simulink model "FullVehicleModel_ABS_ESP"  (R2020a)
settings: Solver=ode23s  StartTime=0.0  StopTime=t_f  MaxStep=0.1  RelTol=1e-3
values from neighbouring files (symbols this model uses):
  acc_US_test = 0.1    [mainVehicleModel.m]
  auxiliary_data = getAuxiliaryDataStruct()    [mainVehicleModel.m]
  curv_akermann = 1/50.    (= 0.02)    [mainVehicleModel.m]
  init_conditions_data = getInitialConditionsDataStruct( V_init )    [mainVehicleModel.m]
  lambda_max = -0.055    [mainVehicleModel.m]
  lambda_min = -0.08    [mainVehicleModel.m]
  maneuver_flag = 4    [mainVehicleModel.m]
  t_brake = t_f+1    (= 111)    [mainVehicleModel.m]
  Tb_max = Fb_max*vehicle_data.rear_wheel.Rr    [mainVehicleModel.m]
  Tb_min = Fb_min*vehicle_data.rear_wheel.Rr    [mainVehicleModel.m]
  V_init = 50    [mainVehicleModel.m]
  vehicle_data = getVehicleDataStruct()    [mainVehicleModel.m]
undefined symbols (not defined in the file or in its folder): k, magnitude, sigbuilder_block
libraries: dspfdesign x1, simulink x1
settings Model: SimulationMode=accelerator  Creator=luca  LastModifiedBy=Pasquale Romano
settings DataIOCC: ReturnWorkspaceOutputs=off
settings DebuggingCC: ArithmeticOperatorsInVariantConditions=warning
settings SFSimCC: SimUseLocalCustomCode=off  CustomCodeUndefinedFunction=UseInterfaceOnly
settings RTWCC: RTWUseLocalCustomCode=off
settings CodeAppCC: StateflowObjectComments=on

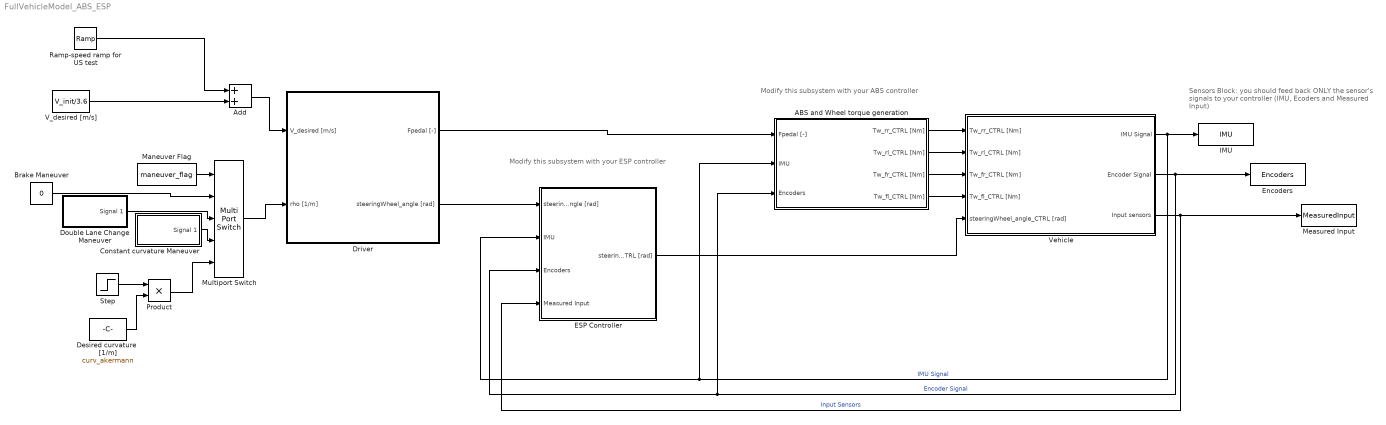
== system FullVehicleModel_ABS_ESP ==
  note: Modify this subsystem with your ABS controller
  note: Modify this subsystem with your ESP
      | controller
  note: Sensors Block: you should feed back ONLY
      | the sensor's signals to your controller
      | (IMU, Ecoders and Measured Input)
  ABS and Wheel torque generation : Subsystem
  Add : Sum
  Brake Maneuver : Constant  Value=0
  Constant curvature Maneuver : Subsystem  Tag=STV Subsys  LoadFcn=sigbuilder_block('load');  StartFcn=sigbuilder_block('start');  StopFcn=sigbuilder_block('stop');  ClipboardFcn=sigbuilder_block('clipboard');  mask(Sigbuilder block){tuvar=[0:10]}
      mask help: Simulink:masks:SigbuilderBlock_MD
      mask init:
      | if ~strcmp(get_param(bdroot(gcbh),'SimulationStatus'),'stopped') tuvar = sigbuilder_block('maskInit'); end
      settings: CopyFcn=sigbuilder_block('copy');  DeleteFcn=sigbuilder_block('delete');  ModelCloseFcn=sigbuilder_block('modelClose');  PreSaveFcn=sigbuilder_block('preSave');  PauseFcn=sigbuilder_block('pause');  ContinueFcn=sigbuilder_block('continue');  NameChangeFcn=sigbuilder_block('namechange');  OpenFcn=sigbuilder_block('open',[0 0 1319 754 ]);  CloseFcn=sigbuilder_block('close');
      mask Display: plot(0, 0, 100, 100,[2, 2, 32, 32, 2], [68, 8, 8, 68, 68],[32, 2], [38, 38], [32, 19, 2],[53, 60, 44], [32, 17, 17, 2],[16, 16, 31, 31]);txt = getActiveGroup(gcbh);text(2, 100, txt,'verticalAlignment', 'top');
  Desired curvature  [1/m] : Constant  Value=curv_akermann
  Double Lane Change Maneuver : Subsystem  Tag=STV Subsys  LoadFcn=sigbuilder_block('load');  StartFcn=sigbuilder_block('start');  StopFcn=sigbuilder_block('stop');  ClipboardFcn=sigbuilder_block('clipboard');  mask(Sigbuilder block){tuvar=[0:10]}
      mask help: Simulink:masks:SigbuilderBlock_MD
      mask init:
      | if ~strcmp(get_param(bdroot(gcbh),'SimulationStatus'),'stopped') tuvar = sigbuilder_block('maskInit'); end
      settings: CopyFcn=sigbuilder_block('copy');  DeleteFcn=sigbuilder_block('delete');  ModelCloseFcn=sigbuilder_block('modelClose');  PreSaveFcn=sigbuilder_block('preSave');  PauseFcn=sigbuilder_block('pause');  ContinueFcn=sigbuilder_block('continue');  NameChangeFcn=sigbuilder_block('namechange');  OpenFcn=sigbuilder_block('open',[0 0 1280 649 ]);  CloseFcn=sigbuilder_block('close');
      mask Display: plot(0, 0, 100, 100,[2, 2, 32, 32, 2], [68, 8, 8, 68, 68],[32, 2], [38, 38], [32, 19, 2],[53, 60, 44], [32, 17, 17, 2],[16, 16, 31, 31]);txt = getActiveGroup(gcbh);text(2, 100, txt,'verticalAlignment', 'top');
  Driver : Subsystem
  ESP Controller : Subsystem
  Encoders : ToWorkspace  VariableName=Encoders  SaveFormat=Timeseries  SampleTime=-1
  IMU : ToWorkspace  VariableName=IMU  SaveFormat=Timeseries  SampleTime=-1
  Maneuver Flag : Constant  Value=maneuver_flag
  Measured Input : ToWorkspace  VariableName=MeasuredInput  SaveFormat=Timeseries  SampleTime=-1
  Multiport Switch : MultiPortSwitch  Inputs=4
  Product : Product
  Ramp-speed ramp for US test : simulink/Sources/Ramp  slope=acc_US_test  start=Tstart_US_test  InitialOutput=0
  Step : Step  SampleTime=0
  V_desired [m/s] : Constant  Value=V_init/3.6
  Vehicle : Subsystem
  wires:
  Driver/1(Fpedal [-]) -> ABS and Wheel torque generation/1(Fpedal [-])
  Driver/2(steeringWheel_angle [rad]) -> ESP Controller/1(steeringWheel_angle [rad])
  Vehicle/1(IMU Signal) -> IMU/1, ABS and Wheel torque generation/2(IMU), ESP Controller/2(IMU)  "IMU Signal"
  Vehicle/2(Encoder Signal) -> Encoders/1, ABS and Wheel torque generation/3(Encoders), ESP Controller/3(Encoders)  "Encoder Signal"
  Vehicle/3(Input sensors) -> Measured Input/1, ESP Controller/4(Measured Input)  "Input Sensors"
  ESP Controller/1(steeringWheel_angle_CTRL [rad]) -> Vehicle/5(steeringWheel_angle_CTRL [rad])
  Double Lane Change Maneuver/1(Signal 1) -> Multiport Switch/3
  Constant curvature Maneuver/1(Signal 1) -> Multiport Switch/4
  Multiport Switch/1 -> Driver/2(rho [1/m])
  Brake Maneuver/1 -> Multiport Switch/2
  Maneuver Flag/1 -> Multiport Switch/1
  ABS and Wheel torque generation/4(Tw_fl_CTRL [Nm]) -> Vehicle/4(Tw_fl_CTRL [Nm])
  ABS and Wheel torque generation/3(Tw_fr_CTRL [Nm]) -> Vehicle/3(Tw_fr_CTRL [Nm])
  ABS and Wheel torque generation/2(Tw_rl_CTRL [Nm]) -> Vehicle/2(Tw_rl_CTRL [Nm])
  ABS and Wheel torque generation/1(Tw_rr_CTRL [Nm]) -> Vehicle/1(Tw_rr_CTRL [Nm])
  Desired curvature  [1/m]/1 -> Product/2
  Step/1 -> Product/1
  Product/1 -> Multiport Switch/5
  Ramp-speed ramp for US test/1 -> Add/1
  V_desired [m/s]/1 -> Add/2
  Add/1 -> Driver/1(V_desired [m/s])

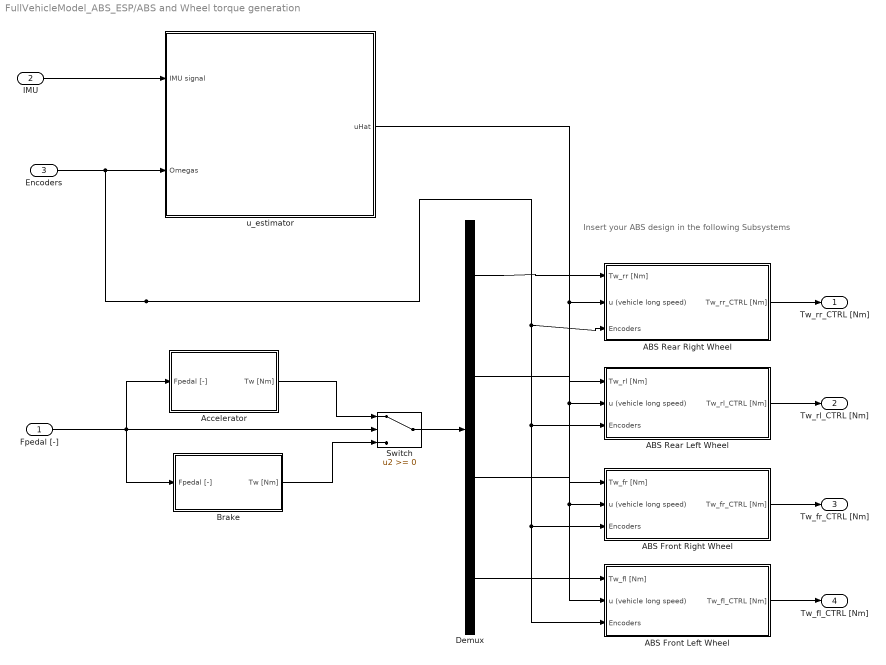
== system FullVehicleModel_ABS_ESP/ABS and Wheel torque generation ==
  note: Insert your ABS design in the
      | following Subsystems
  Fpedal [-] : Inport
  IMU : Inport  Port=2
  Encoders : Inport  Port=3
  ABS Front Left Wheel : Subsystem
  ABS Front Right Wheel : Subsystem
  ABS Rear Left Wheel : Subsystem
  ABS Rear Right Wheel : Subsystem
  Accelerator : Subsystem
  Brake : Subsystem
  Demux : Demux
  Switch : Switch
  u_estimator : Subsystem
  Tw_rr_CTRL [Nm] : Outport  VectorParamsAs1DForOutWhenUnconnected=off
  Tw_rl_CTRL [Nm] : Outport  Port=2  VectorParamsAs1DForOutWhenUnconnected=off
  Tw_fr_CTRL [Nm] : Outport  Port=3  VectorParamsAs1DForOutWhenUnconnected=off
  Tw_fl_CTRL [Nm] : Outport  Port=4  VectorParamsAs1DForOutWhenUnconnected=off
  wires:
  Demux/2 -> ABS Rear Left Wheel/1(Tw_rl [Nm])
  Switch/1 -> Demux/1
  Demux/1 -> ABS Rear Right Wheel/1(Tw_rr [Nm])
  Fpedal [-]/1 -> Brake/1(Fpedal [-]), Accelerator/1(Fpedal [-]), Switch/2
  ABS Rear Right Wheel/1(Tw_rr_CTRL [Nm]) -> Tw_rr_CTRL [Nm]/1
  Encoders/1 -> u_estimator/2(Omegas), ABS Rear Right Wheel/3(Encoders), ABS Front Left Wheel/3(Encoders), ABS Front Right Wheel/3(Encoders), ABS Rear Left Wheel/3(Encoders)
  ABS Rear Left Wheel/1(Tw_rl_CTRL [Nm]) -> Tw_rl_CTRL [Nm]/1
  Demux/3 -> ABS Front Right Wheel/1(Tw_fr [Nm])
  ABS Front Right Wheel/1(Tw_fr_CTRL [Nm]) -> Tw_fr_CTRL [Nm]/1
  Demux/4 -> ABS Front Left Wheel/1(Tw_fl [Nm])
  ABS Front Left Wheel/1(Tw_fl_CTRL [Nm]) -> Tw_fl_CTRL [Nm]/1
  Accelerator/1(Tw [Nm]) -> Switch/1
  Brake/1(Tw [Nm]) -> Switch/3
  IMU/1 -> u_estimator/1(IMU signal)
  u_estimator/1(uHat) -> ABS Front Right Wheel/2("u (vehicle long speed) "), ABS Front Left Wheel/2("u (vehicle long speed) "), ABS Rear Left Wheel/2("u (vehicle long speed) "), ABS Rear Right Wheel/2("u (vehicle long speed) ")

== system FullVehicleModel_ABS_ESP/Constant curvature Maneuver ==
  Demux : Demux  Tag=STV Demux  Outputs=1
      settings: DisplayOption=none
  FromWs : FromWorkspace  Tag=STV FromWs  VariableName=tuvar
      SigBuilderData=|
      | common.afterFinalStr = 'Extrapolate'
      | common.sampleTime = 0
      | dataSet.timeRange = [0 20]
      | dataSet.name = 'Group 1'
      | sbobj.Groups.Name = 'Group 1'
      | sbobj.Groups.Signals.Name = 'Signal 1'
      | sbobj.Groups.Signals.XData = [0 0.98 0.98 20]
      | sbobj.Groups.Signals.YData = [0 0 0.4 0.4]
      | sbobj.Groups.TimeRange = [0 20]
  Signal 1 : Outport  Tag=STV Outport  VectorParamsAs1DForOutWhenUnconnected=off
  wires:
  Demux/1 -> Signal 1/1
  FromWs/1 -> Demux/1

== system FullVehicleModel_ABS_ESP/Double Lane Change Maneuver ==
  Demux : Demux  Tag=STV Demux  Outputs=1
      settings: DisplayOption=none
  FromWs : FromWorkspace  Tag=STV FromWs  VariableName=tuvar
      SigBuilderData=|
      | common.afterFinalStr = 'Extrapolate'
      | common.sampleTime = 0
      | dataSet.timeRange = [0 10]
      | dataSet.name = 'Group 1'
      | sbobj.Groups.Name = 'Group 1'
      | sbobj.Groups.Signals.Name = 'Signal 1'
      | sbobj.Groups.Signals.XData = [0 1 1 1.5 1.5 1.6 1.6 2.1 2.1 3 3 3.5 3.5 3.7 3.7 4.2 4.2 10]
      | sbobj.Groups.Signals.YData = [0 0 0.5 0.5 0 0 -0.504 -0.504 0 0 -0.5 -0.5 0 0 0.5 0.5 0 0]
  Signal 1 : Outport  Tag=STV Outport  VectorParamsAs1DForOutWhenUnconnected=off
  wires:
  FromWs/1 -> Demux/1
  Demux/1 -> Signal 1/1

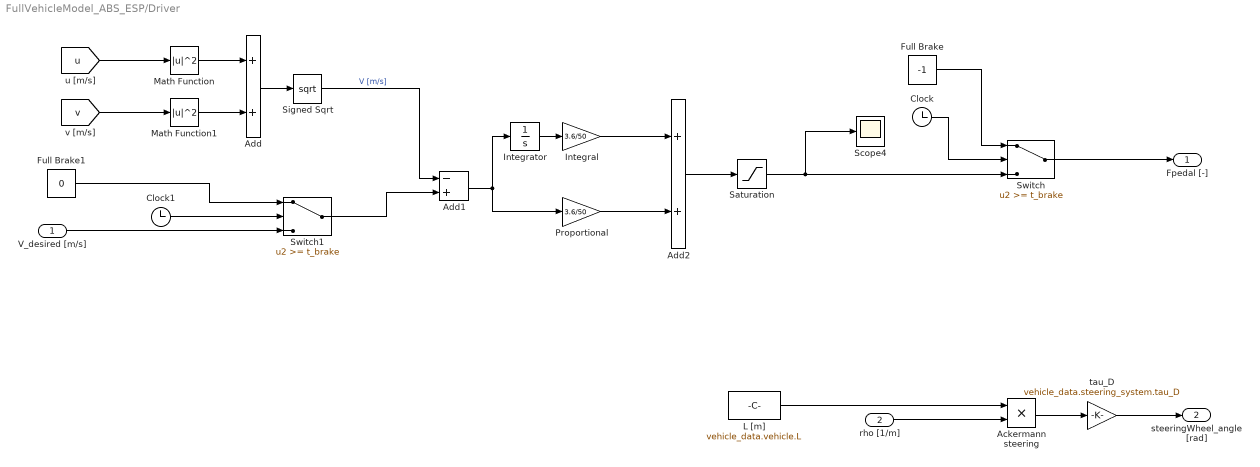
== system FullVehicleModel_ABS_ESP/Driver ==
  V_desired [m/s] : Inport
  rho [1/m] : Inport  Port=2
  Ackermann steering : Product  Inputs=**
  Add : Sum
  Add1 : Sum  Inputs=-+
  Add2 : Sum
  Clock : Clock
  Clock1 : Clock
  Full Brake : Constant  Value=-1
  Full Brake1 : Constant  Value=0
  Integral : Gain  Gain=3.6/50
  Integrator : Integrator
  L [m] : Constant  Value=vehicle_data.vehicle.L
  Math Function : Math  Operator=magnitude^2  SignedPower=on  SaturateOnIntegerOverflow=on
  Math Function1 : Math  Operator=magnitude^2  SignedPower=on  SaturateOnIntegerOverflow=on
  Proportional : Gain  Gain=3.6/50
  Saturation : Saturate  UpperLimit=1  LowerLimit=-1
  Scope4 : Scope
  Signed Sqrt : Sqrt  SaturateOnIntegerOverflow=on
  Switch : Switch  Threshold=t_brake
  Switch1 : Switch  Threshold=t_brake
  tau_D : Gain  Gain=vehicle_data.steering_system.tau_D
  Fpedal [-] : Outport  VectorParamsAs1DForOutWhenUnconnected=off
  steeringWheel_angle [rad] : Outport  Port=2  VectorParamsAs1DForOutWhenUnconnected=off
  wires:
  Proportional/1 -> Add2/2
  Add2/1 -> Saturation/1
  Integrator/1 -> Integral/1
  L [m]/1 -> Ackermann steering/1
  Add/1 -> Signed Sqrt/1
  Math Function1/1 -> Add/2
  Add1/1 -> Integrator/1, Proportional/1
  Signed Sqrt/1 -> Add1/1  "V [m/s]"
  Ackermann steering/1 -> tau_D/1
  Math Function/1 -> Add/1
  rho [1/m]/1 -> Ackermann steering/2
  Integral/1 -> Add2/1
  [u] -> Math Function/1
  [v] -> Math Function1/1
  V_desired [m/s]/1 -> Switch1/3
  Saturation/1 -> Switch/3, Scope4/1
  Full Brake1/1 -> Switch1/1
  Clock1/1 -> Switch1/2
  Full Brake/1 -> Switch/1
  Clock/1 -> Switch/2
  Switch/1 -> Fpedal [-]/1
  Switch1/1 -> Add1/2
  tau_D/1 -> steeringWheel_angle [rad]/1

== system FullVehicleModel_ABS_ESP/ESP Controller ==
  steeringWheel_angle [rad] : Inport
  IMU : Inport  Port=2
  Encoders : Inport  Port=3
  Measured Input : Inport  Port=4
  Terminator : Terminator
  Terminator1 : Terminator
  Terminator2 : Terminator
  steeringWheel_angle_CTRL [rad] : Outport  VectorParamsAs1DForOutWhenUnconnected=off
  wires:
  steeringWheel_angle [rad]/1 -> steeringWheel_angle_CTRL [rad]/1
  IMU/1 -> Terminator/1
  Encoders/1 -> Terminator1/1
  Measured Input/1 -> Terminator2/1

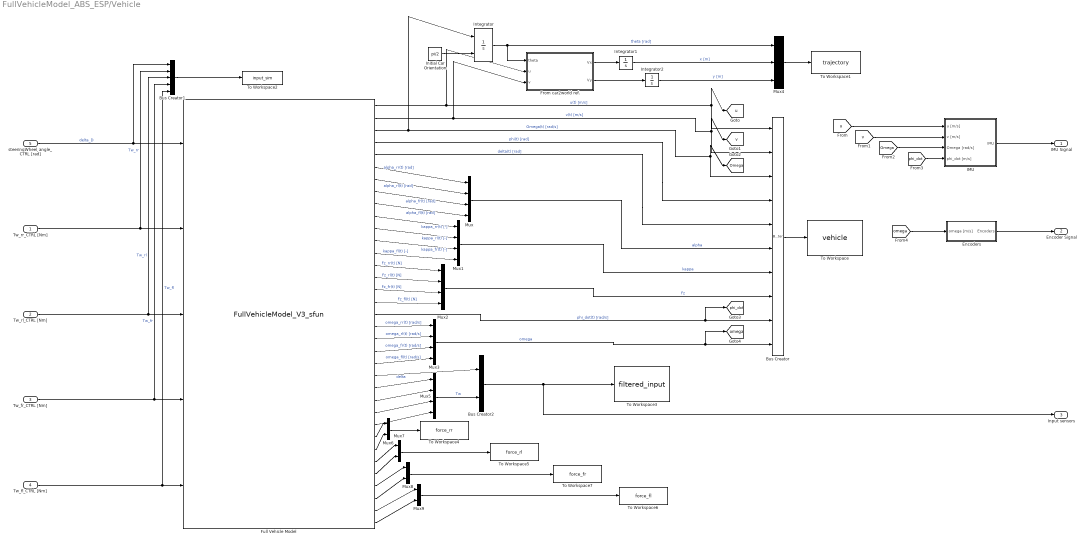
== system FullVehicleModel_ABS_ESP/Vehicle ==
  Tw_rr_CTRL [Nm] : Inport
  Tw_rl_CTRL [Nm] : Inport  Port=2
  Tw_fr_CTRL [Nm] : Inport  Port=3
  Tw_fl_CTRL [Nm] : Inport  Port=4
  steeringWheel_angle_CTRL [rad] : Inport  Port=5
  Bus Creator : BusCreator  Inputs=10
  Bus Creator1 : BusCreator  Inputs=5
  Bus Creator2 : BusCreator  Inputs=2
  Encoders : Subsystem
  "From car2world ref. " : Subsystem
  Full Vehicle Model : M-S-Function  FunctionName=FullVehicleModel_V3_sfun  Parameters=vehicle_data, init_conditions_data, auxiliary_data  mask(Matlab S-function:FullVehicleModel_V3_sfun){vehicle_data=vehicle_data, init_conditions_data=init_conditions_data, auxiliary_data=auxiliary_data}
      mask prompts: vehicle_data "Vehicle data structure"; init_conditions_data "Initial conditions structure"; auxiliary_data "Auxiliary data"
      mask help: This is a level-2 MATLAB file S-function that implements full vehicle dynamics at high and low speeds. This includes the vertical and lateral dynamics, together with wheel dynamics (wheels speed, lateral and longitudinal slip) and roll dynamics.
      mask Display:
      | port_label('input', 1, 'delta_D [rad]');
      | port_label('input', 2, 'Tw_rr [Nm]');
      | port_label('input', 3, 'Tw_rl [Nm]');
      | port_label('input', 4, 'Tw_fr [Nm]');
      | port_label('input', 5, 'Tw_fl [Nm]');
      | 
      | % x(1)  = u(t)        -> Longitudinal vehicle velocity
      | port_label('output', 1, 'u [m/s]');
      | % x(2)  = v(t)        -> Lateral vehicle velocity
      | port_label('output', 2, 'v [m/s]');
      | % x(3)  = Omega(t)    -> Yaw rate
      | port_label('output', 3, 'Omega [rad/s]');
      | % x(4)  = phi(t)      -> Roll angle
      | port_label('output', 4, 'phi [rad]');
      | % x(5)  = delta(t)    -> Steering angle
      | port_label('output', 5, 'delta [rad]');
      | % x(6)  = alpha_rr(t) -> Side slip angle, rear right wheel
      | port_label('output', 6, 'alpha_rr [-]');
      | % x(7)  = alpha_rl(t) -> Side slip angle, rear left wheel
      | port_label('output', 7, 'alpha_rl [-]');
      | % x(8)  = alpha_fr(t) -> Side slip angle, front right wheel
      | port_label('output', 8, 'alpha_fr [-]');
      | % x(9)  = alpha_fl(t) -> Side slip angle, front left wheel
      | port_label('output', 9, 'alpha_fl [-]');
      | % x(10) = kappa_rr(t) -> Longitudinal slip, rear right wheel
      | port_label('output', 10, 'kappa_rr [-]');
      | % x(11) = kappa_rl(t) -> Longitudinal slip, rear left wheel
      | port_label('output', 11, 'kappa_rl [-]');
      | % x(12) = kappa_fr(t) -> Longitudinal slip, front right wheel
      | port_label('output', 12, 'kappa_fr [-]');
      | % x(13) = kappa_fl(t) -> Longitudinal slip, front left wheel
      | port_label('output', 13, 'kappa_fl [-]');
      | % x(14) = Fz_rr(t)    -> Vertical load, rear right wheel
      | port_label('output', 14, 'Fz_rr [N]');
      | % x(15) = Fz_rl(t)    -> Vertical load, rear rear left wheel
      | port_label('output', 15, 'Fz_rl [N]');
      | % x(16) = Fz_fr(t)    -> Vertical load, front right wheel
      | port_label('output', 16, 'Fz_fr [N]');
      | % x(17) = Fz_fl(t)    -> Vertical load, front left wheel
      | port_label('output', 17, 'Fz_fl [N]');
      | % x(18) = phi_dot(t)  -> Roll rate
      | port_label('output', 18, 'phi_dot [rad/s]');
      | % x(19) = omega_rr(t) -> angular velocity rear right wheel
      | port_label('output', 19, 'omega_rr [rad/s]');
      | % x(20) = omega_rl(t) -> angular velocity rear left wheel
      | port_label('output', 20, 'omega_rl [rad/s]');
      | % x(21) = omega_fr(t) -> angular velocity front right wheel
      | port_label('output', 21, 'omega_fr [rad/s]');
      | % x(22) = omega_fl(t) -> angular velocity front left wheel
      | port_label('output', 22, 'omega_fl [rad/s]');
      | % x(23) = delta(t) -> real steer angle
      | port_label('output', 23, 'delta [rad]');
      | % x(24:27) = Tw(t) -> Filtered wheel torque
      | port_label('output', 24, 'Tw_rr [Nm]');
      | port_label('output', 25, 'Tw_rl [Nm]');
      | port_label('output', 26, 'Tw_fr [Nm]');
      | port_label('output', 27, 'Tw_fl [Nm]');
      | 
      | % Wheel forces
      | % Rear Right
      | port_label('output', 28, 'Fx_rr [N]');
      | port_label('output', 29, 'Fy_rr [N]');
      | % Rear Left
      | port_label('output', 30, 'Fx_rl [N]');
      | port_label('output', 31, 'Fy_rl [N]');
      | % Front Right
      | port_label('output', 32, 'Fx_fr [N]');
      | port_label('output', 33, 'Fy_fr [N]');
      | % Front Left
      | port_label('output', 34, 'Fx_fl [N]');
      | port_label('output', 35, 'Fy_fl [N]');
  IMU : Subsystem
  Initial Car Orientation : Constant  Value=pi/2
  Integrator : Integrator  InitialConditionSource=external
  Integrator1 : Integrator
  Integrator2 : Integrator
  Mux{,1..3,5} (5 alike) : Mux
  Mux4 : Mux  Inputs=3
  Mux{6..9} (4 alike) : Mux  Inputs=2
  To Workspace : ToWorkspace  VariableName=vehicle  SaveFormat=Timeseries  SampleTime=-1
  To Workspace1 : ToWorkspace  VariableName=trajectory  SaveFormat=Timeseries  SampleTime=-1
  To Workspace2 : ToWorkspace  VariableName=input_sim  SaveFormat=Timeseries  SampleTime=-1
  To Workspace3 : ToWorkspace  VariableName=filtered_input  SaveFormat=Timeseries  SampleTime=-1
  To Workspace4 : ToWorkspace  VariableName=force_rr  SaveFormat=Timeseries  SampleTime=-1
  To Workspace5 : ToWorkspace  VariableName=force_rl  SaveFormat=Timeseries  SampleTime=-1
  To Workspace6 : ToWorkspace  VariableName=force_fl  SaveFormat=Timeseries  SampleTime=-1
  To Workspace7 : ToWorkspace  VariableName=force_fr  SaveFormat=Timeseries  SampleTime=-1
  IMU Signal : Outport  VectorParamsAs1DForOutWhenUnconnected=off
  Encoder Signal : Outport  Port=2  VectorParamsAs1DForOutWhenUnconnected=off
  Input sensors : Outport  Port=3  VectorParamsAs1DForOutWhenUnconnected=off
  tag scope: Omega=global, omega=global, phi_dot=global, u=global, v=global
  wires:
  Mux5/1 -> Bus Creator2/2  "Tw"
  Full Vehicle Model/4 -> Bus Creator/4  "phi(t) [rad]"
  Integrator/1 -> "From car2world ref. "/1(theta), Mux4/1  "theta [rad]"
  Mux8/1 -> To Workspace7/1
  Full Vehicle Model/32 -> Mux8/1
  Mux2/1 -> Bus Creator/8  "Fz"
  "From car2world ref. "/1(Vx) -> Integrator1/1
  Full Vehicle Model/28 -> Mux6/1
  Full Vehicle Model/35 -> Mux9/2
  Full Vehicle Model/19 -> Mux3/1  "omega_rr(t) [rad/s]"
  Mux7/1 -> To Workspace5/1
  Mux9/1 -> To Workspace6/1
  Bus Creator/1 -> To Workspace/1
  Full Vehicle Model/6 -> Mux/1  "alpha_rr(t) [rad]"
  Full Vehicle Model/2 -> [v], Bus Creator/2, "From car2world ref. "/3(v)  "v(t) [m/s]"
  Full Vehicle Model/7 -> Mux/2  "alpha_rl(t) [rad]"
  Full Vehicle Model/12 -> Mux1/3  "kappa_fr(t) [-]"
  Full Vehicle Model/20 -> Mux3/2  "omega_rl(t) [rad/s]"
  Full Vehicle Model/16 -> Mux2/3  "Fz_fr(t) [N]"
  Full Vehicle Model/9 -> Mux/4  "alpha_fl(t) [rad]"
  Full Vehicle Model/10 -> Mux1/1  "kappa_rr(t) [-]"
  Full Vehicle Model/11 -> Mux1/2  "kappa_rl(t) [-]"
  Full Vehicle Model/31 -> Mux7/2
  Full Vehicle Model/26 -> Mux5/3
  Full Vehicle Model/24 -> Mux5/1
  Full Vehicle Model/23 -> Bus Creator2/1  "delta"
  Full Vehicle Model/8 -> Mux/3  "alpha_fr(t) [rad]"
  Initial Car Orientation/1 -> Integrator/2
  Full Vehicle Model/22 -> Mux3/4  "omega_fl(t) [rad/s]"
  Bus Creator2/1 -> Input sensors/1, To Workspace3/1
  Full Vehicle Model/29 -> Mux6/2
  Full Vehicle Model/5 -> Bus Creator/5  "delta(t) [rad]"
  Full Vehicle Model/21 -> Mux3/3  "omega_fr(t) [rad/s]"
  Full Vehicle Model/3 -> [Omega], Bus Creator/3, Integrator/1  "Omega(t) [rad/s]"
  Mux3/1 -> Bus Creator/10, [omega]  "omega"
  Full Vehicle Model/1 -> [u], Bus Creator/1, "From car2world ref. "/2(u)  "u(t) [m/s]"
  Full Vehicle Model/13 -> Mux1/4  "kappa_fl(t) [-]"
  Mux4/1 -> To Workspace1/1
  Bus Creator1/1 -> To Workspace2/1
  steeringWheel_angle_CTRL [rad]/1 -> Bus Creator1/1, Full Vehicle Model/1  "delta_D"
  Full Vehicle Model/18 -> Bus Creator/9, [phi_dot]  "phi_dot(t) [rad/s]"
  Full Vehicle Model/30 -> Mux7/1
  Integrator2/1 -> Mux4/3  "y [m]"
  Mux6/1 -> To Workspace4/1
  Mux/1 -> Bus Creator/6  "alpha"
  Full Vehicle Model/27 -> Mux5/4
  Full Vehicle Model/17 -> Mux2/4  "Fz_fl(t) [N]"
  Integrator1/1 -> Mux4/2  "x [m]"
  "From car2world ref. "/2(Vy) -> Integrator2/1
  Full Vehicle Model/14 -> Mux2/1  "Fz_rr(t) [N]"
  Mux1/1 -> Bus Creator/7  "kappa"
  Full Vehicle Model/25 -> Mux5/2
  Full Vehicle Model/15 -> Mux2/2  "Fz_rl(t) [N]"
  Full Vehicle Model/34 -> Mux9/1
  Full Vehicle Model/33 -> Mux8/2
  Tw_rr_CTRL [Nm]/1 -> Bus Creator1/2, Full Vehicle Model/2  "Tw_rr"
  Tw_rl_CTRL [Nm]/1 -> Bus Creator1/3, Full Vehicle Model/3  "Tw_rl"
  Tw_fr_CTRL [Nm]/1 -> Bus Creator1/4, Full Vehicle Model/4  "Tw_fr"
  Tw_fl_CTRL [Nm]/1 -> Bus Creator1/5, Full Vehicle Model/5  "Tw_fl"
  [u] -> IMU/1(u [m/s])
  [v] -> IMU/2(v [m/s])
  IMU/1(IMU) -> IMU Signal/1
  [Omega] -> IMU/3(Omega [rad/s])
  [phi_dot] -> IMU/4(phi_dot [m/s])
  [omega] -> Encoders/1(omega [m/s])
  Encoders/1(Encoders) -> Encoder Signal/1

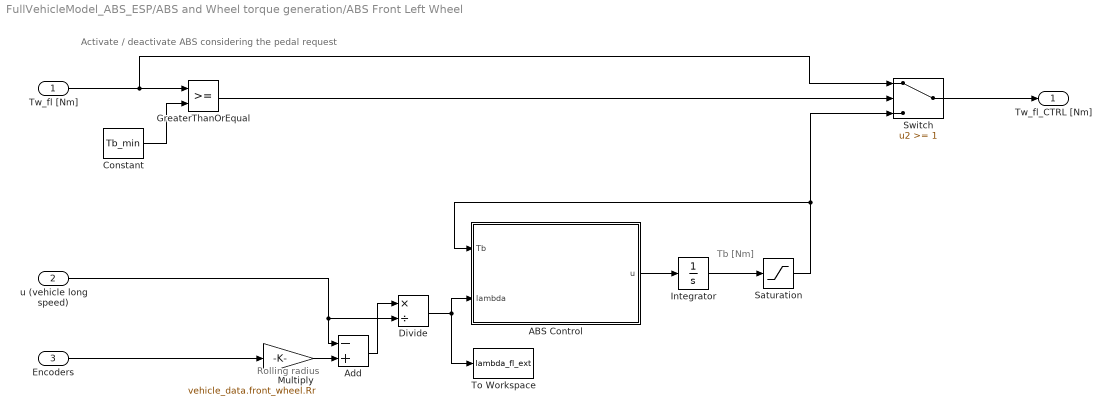
== system FullVehicleModel_ABS_ESP/ABS and Wheel torque generation/ABS Front Left Wheel ==
  note: Activate / deactivate ABS considering the pedal request
  note: Rolling radius
  note: Tb [Nm]
  Tw_fl [Nm] : Inport
  "u (vehicle long speed) " : Inport  Port=2
  Encoders : Inport  Port=3
  ABS Control : Stateflow chart  TreatAsAtomicUnit=on
  Add : Sum  Inputs=-+
  Constant : Constant  Value=Tb_min
  Divide : Product  Inputs=*/
  GreaterThanOrEqual : RelationalOperator  OutDataTypeStr=boolean  RndMeth=Simplest
  Integrator : Integrator
  Multiply : Gain  Gain=vehicle_data.front_wheel.Rr
  Saturation : Saturate  UpperLimit=3e3  LowerLimit=-3e3
  Switch : Switch  Threshold=1
  To Workspace : ToWorkspace  VariableName=lambda_fl_ext  SampleTime=-1
      settings: Save2DSignal=2-D array (concatenate along first dimension)
  Tw_fl_CTRL [Nm] : Outport  VectorParamsAs1DForOutWhenUnconnected=off
  wires:
  ABS Control/1(u) -> Integrator/1
  Saturation/1 -> Switch/3, ABS Control/1(Tb)
  Divide/1 -> To Workspace/1, ABS Control/2(lambda)
  Integrator/1 -> Saturation/1
  Constant/1 -> GreaterThanOrEqual/2
  "u (vehicle long speed) "/1 -> Add/1, Divide/2
  Multiply/1 -> Add/2
  Add/1 -> Divide/1
  Tw_fl [Nm]/1 -> GreaterThanOrEqual/1, Switch/1
  GreaterThanOrEqual/1 -> Switch/2
  Switch/1 -> Tw_fl_CTRL [Nm]/1
  Encoders/1 -> Multiply/1

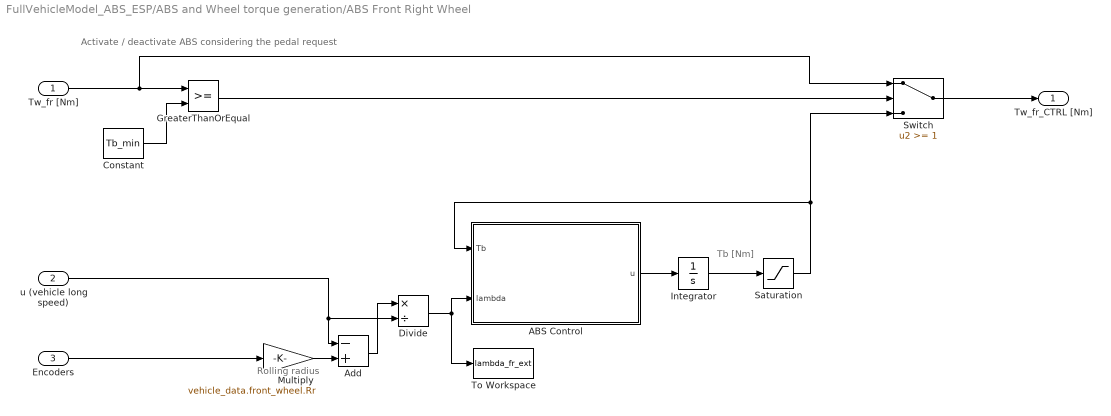
== system FullVehicleModel_ABS_ESP/ABS and Wheel torque generation/ABS Front Right Wheel ==
  note: Activate / deactivate ABS considering the pedal request
  note: Rolling radius
  note: Tb [Nm]
  Tw_fr [Nm] : Inport
  "u (vehicle long speed) " : Inport  Port=2
  Encoders : Inport  Port=3
  ABS Control : Stateflow chart  TreatAsAtomicUnit=on
  Add : Sum  Inputs=-+
  Constant : Constant  Value=Tb_min
  Divide : Product  Inputs=*/
  GreaterThanOrEqual : RelationalOperator  OutDataTypeStr=boolean  RndMeth=Simplest
  Integrator : Integrator
  Multiply : Gain  Gain=vehicle_data.front_wheel.Rr
  Saturation : Saturate  UpperLimit=3e3  LowerLimit=-3e3
  Switch : Switch  Threshold=1
  To Workspace : ToWorkspace  VariableName=lambda_fr_ext  SampleTime=-1
      settings: Save2DSignal=2-D array (concatenate along first dimension)
  Tw_fr_CTRL [Nm] : Outport  VectorParamsAs1DForOutWhenUnconnected=off
  wires:
  ABS Control/1(u) -> Integrator/1
  Saturation/1 -> Switch/3, ABS Control/1(Tb)
  Divide/1 -> To Workspace/1, ABS Control/2(lambda)
  Integrator/1 -> Saturation/1
  Constant/1 -> GreaterThanOrEqual/2
  "u (vehicle long speed) "/1 -> Add/1, Divide/2
  Multiply/1 -> Add/2
  Add/1 -> Divide/1
  Tw_fr [Nm]/1 -> GreaterThanOrEqual/1, Switch/1
  GreaterThanOrEqual/1 -> Switch/2
  Switch/1 -> Tw_fr_CTRL [Nm]/1
  Encoders/1 -> Multiply/1

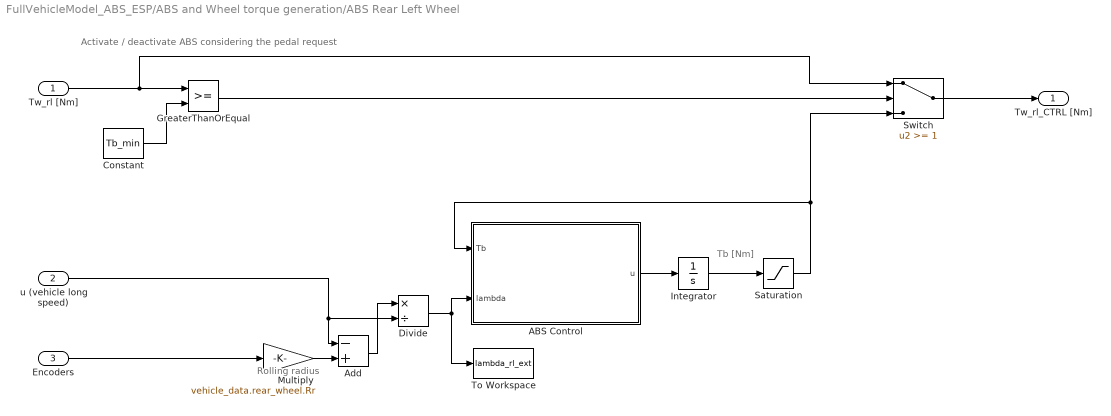
== system FullVehicleModel_ABS_ESP/ABS and Wheel torque generation/ABS Rear Left Wheel ==
  note: Activate / deactivate ABS considering the pedal request
  note: Rolling radius
  note: Tb [Nm]
  Tw_rl [Nm] : Inport
  "u (vehicle long speed) " : Inport  Port=2
  Encoders : Inport  Port=3
  ABS Control : Stateflow chart  TreatAsAtomicUnit=on
  Add : Sum  Inputs=-+
  Constant : Constant  Value=Tb_min
  Divide : Product  Inputs=*/
  GreaterThanOrEqual : RelationalOperator  OutDataTypeStr=boolean  RndMeth=Simplest
  Integrator : Integrator
  Multiply : Gain  Gain=vehicle_data.rear_wheel.Rr
  Saturation : Saturate  UpperLimit=3e3  LowerLimit=-3e3
  Switch : Switch  Threshold=1
  To Workspace : ToWorkspace  VariableName=lambda_rl_ext  SampleTime=-1
      settings: Save2DSignal=2-D array (concatenate along first dimension)
  Tw_rl_CTRL [Nm] : Outport  VectorParamsAs1DForOutWhenUnconnected=off
  wires:
  ABS Control/1(u) -> Integrator/1
  Saturation/1 -> Switch/3, ABS Control/1(Tb)
  Divide/1 -> To Workspace/1, ABS Control/2(lambda)
  Integrator/1 -> Saturation/1
  Constant/1 -> GreaterThanOrEqual/2
  "u (vehicle long speed) "/1 -> Add/1, Divide/2
  Multiply/1 -> Add/2
  Add/1 -> Divide/1
  Tw_rl [Nm]/1 -> GreaterThanOrEqual/1, Switch/1
  GreaterThanOrEqual/1 -> Switch/2
  Switch/1 -> Tw_rl_CTRL [Nm]/1
  Encoders/1 -> Multiply/1

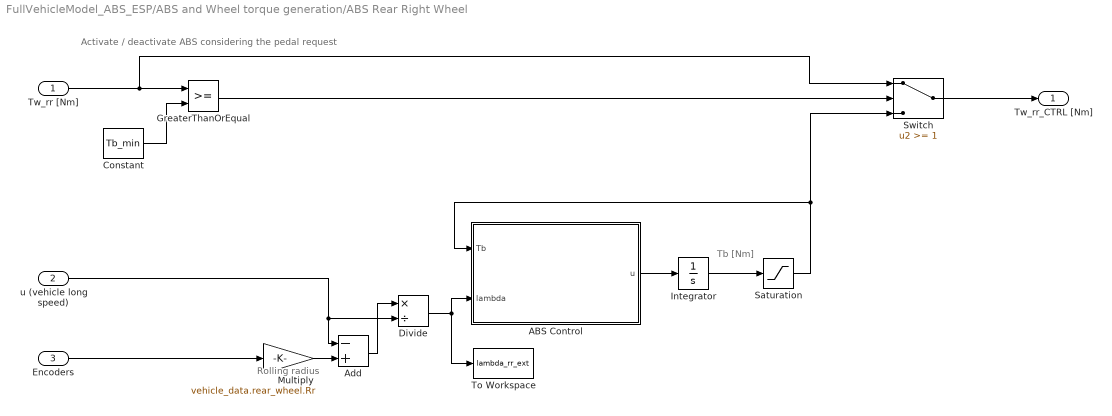
== system FullVehicleModel_ABS_ESP/ABS and Wheel torque generation/ABS Rear Right Wheel ==
  note: Activate / deactivate ABS considering the pedal request
  note: Tb [Nm]
  note: Rolling radius
  Tw_rr [Nm] : Inport
  "u (vehicle long speed) " : Inport  Port=2
  Encoders : Inport  Port=3
  ABS Control : Stateflow chart  TreatAsAtomicUnit=on
  Add : Sum  Inputs=-+
  Constant : Constant  Value=Tb_min
  Divide : Product  Inputs=*/
  GreaterThanOrEqual : RelationalOperator  OutDataTypeStr=boolean  RndMeth=Simplest
  Integrator : Integrator
  Multiply : Gain  Gain=vehicle_data.rear_wheel.Rr
  Saturation : Saturate  UpperLimit=3e3  LowerLimit=-3e3
  Switch : Switch  Threshold=1
  To Workspace : ToWorkspace  VariableName=lambda_rr_ext  SampleTime=-1
      settings: Save2DSignal=2-D array (concatenate along first dimension)
  Tw_rr_CTRL [Nm] : Outport  VectorParamsAs1DForOutWhenUnconnected=off
  wires:
  Switch/1 -> Tw_rr_CTRL [Nm]/1
  Constant/1 -> GreaterThanOrEqual/2
  GreaterThanOrEqual/1 -> Switch/2
  "u (vehicle long speed) "/1 -> Add/1, Divide/2
  Encoders/1 -> Multiply/1
  Saturation/1 -> Switch/3, ABS Control/1(Tb)
  ABS Control/1(u) -> Integrator/1
  Multiply/1 -> Add/2
  Tw_rr [Nm]/1 -> GreaterThanOrEqual/1, Switch/1
  Add/1 -> Divide/1
  Divide/1 -> To Workspace/1, ABS Control/2(lambda)
  Integrator/1 -> Saturation/1

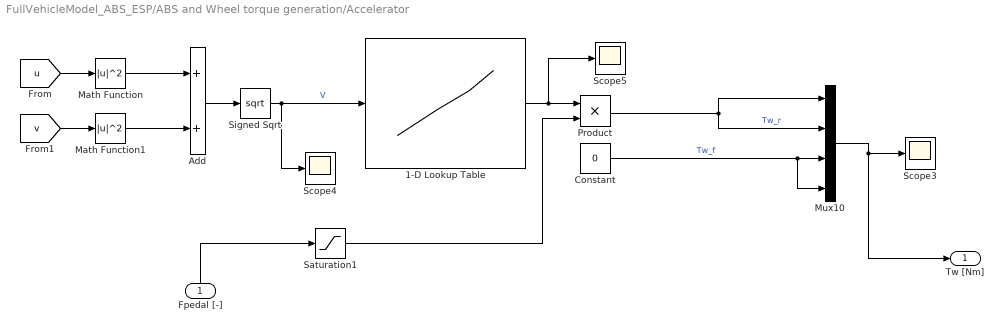
== system FullVehicleModel_ABS_ESP/ABS and Wheel torque generation/Accelerator ==
  Fpedal [-] : Inport
  1-D Lookup Table : Lookup_n-D  NumberOfTableDimensions=1  BreakpointsForDimension1=linspace(0,250/3.6,31)  Table=|  InternalRulePriority=Speed  RndMeth=Simplest  InputSameDT=on
      | 500*[0.442662657646371
      | 0.537281800718283
      | 0.631900943790195
      | 0.726520086862107
      | 0.821139229934018
      | 0.859929256634989
      | 0.897666213627126
      | 0.918905078514199
      | 0.939980602614386
      | 0.959177707665377
      | 0.977316148834879
      | 0.987691054873465
      | 0.996795820900055
      | 1
      | 0.995733117962017
      | 0.989286574404060
      | 0.982840030846103
      | 0.974205033220170
      | 0.965525373266320
      | 0.956088102993640
      | 0.944254781591915
      | 0.930421573540466
      | 0.913474919507860
      | 0.895654110637824
      | 0.877209833235892
      | 0.858765555833960
      | 0.840321278432028
      | 0.817183521078455
      | 0.778999480858075
      | 0.389499740429037
      | 0]
  Add : Sum
  Constant : Constant  Value=0
  Math Function : Math  Operator=magnitude^2  SignedPower=on  SaturateOnIntegerOverflow=on
  Math Function1 : Math  Operator=magnitude^2  SignedPower=on  SaturateOnIntegerOverflow=on
  Mux10 : Mux
  Product : Product
  Saturation1 : Saturate  UpperLimit=1  LowerLimit=0
  Scope3 : Scope
  Scope4 : Scope
  Scope5 : Scope
  Signed Sqrt : Sqrt  SaturateOnIntegerOverflow=on
  Tw [Nm] : Outport  VectorParamsAs1DForOutWhenUnconnected=off
  wires:
  1-D Lookup Table/1 -> Scope5/1, Product/1
  Fpedal [-]/1 -> Saturation1/1
  Constant/1 -> Mux10/4, Mux10/3  "Tw_f"
  [v] -> Math Function1/1
  Signed Sqrt/1 -> Scope4/1, 1-D Lookup Table/1  "V"
  [u] -> Math Function/1
  Math Function/1 -> Add/1
  Product/1 -> Mux10/2, Mux10/1  "Tw_r"
  Mux10/1 -> Tw [Nm]/1, Scope3/1
  Saturation1/1 -> Product/2
  Add/1 -> Signed Sqrt/1
  Math Function1/1 -> Add/2

== system FullVehicleModel_ABS_ESP/ABS and Wheel torque generation/Brake ==
  Fpedal [-] : Inport
  Front Brake ratio : Gain  Gain=0.3
  Max Brake Torque : Gain  Gain=1500
  Mux11 : Mux
  Rate Limiter : RateLimiter  RisingSlewLimit=1e5  FallingSlewLimit=-10000  SampleTimeMode=inherited
  Rear Brake ratio : Gain  Gain=0.7
  Saturation : Saturate  UpperLimit=0  LowerLimit=-1
  Tw [Nm] : Outport  VectorParamsAs1DForOutWhenUnconnected=off
  wires:
  Saturation/1 -> Max Brake Torque/1
  Fpedal [-]/1 -> Saturation/1
  Mux11/1 -> Tw [Nm]/1
  Front Brake ratio/1 -> Mux11/4, Mux11/3
  Rear Brake ratio/1 -> Mux11/2, Mux11/1
  Max Brake Torque/1 -> Rate Limiter/1
  Rate Limiter/1 -> Rear Brake ratio/1, Front Brake ratio/1

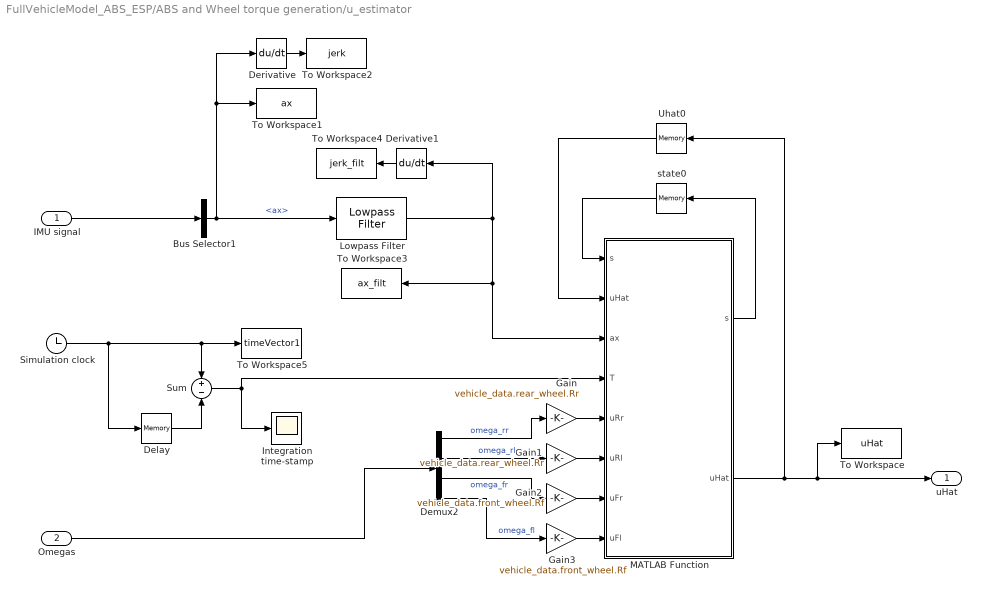
== system FullVehicleModel_ABS_ESP/ABS and Wheel torque generation/u_estimator ==
  IMU signal : Inport
  Omegas : Inport  Port=2
  Bus Selector1 : BusSelector  OutputSignals=ax
  Delay : Memory  InheritSampleTime=on
  Demux2 : Demux
  Derivative : Derivative
  Derivative1 : Derivative
  Gain : Gain  Gain=vehicle_data.rear_wheel.Rr
  Gain1 : Gain  Gain=vehicle_data.rear_wheel.Rr
  Gain2 : Gain  Gain=vehicle_data.front_wheel.Rf
  Gain3 : Gain  Gain=vehicle_data.front_wheel.Rf
  Integration time-stamp : Scope
  Lowpass Filter : dspfdesign/Lowpass Filter  FilterType=FIR  DesignForMinimumOrder=off  FilterOrder=12  PassbandFrequency=10  StopbandFrequency=14  PassbandRipple=0.1  StopbandAttenuation=60  InheritSampleRate=off  SampleRate=44100  SimulateUsing=Interpreted execution  roundingMode=Floor  coeffsDataTypeStr=fixdt(1,16)
  MATLAB Function : MATLAB Function  TreatAsAtomicUnit=on
  Simulation clock : Clock
  Sum : Sum  Inputs=+-
  To Workspace : ToWorkspace  VariableName=uHat  SampleTime=-1
      settings: Save2DSignal=2-D array (concatenate along first dimension)
  To Workspace1 : ToWorkspace  VariableName=ax  SampleTime=-1
      settings: Save2DSignal=2-D array (concatenate along first dimension)
  To Workspace2 : ToWorkspace  VariableName=jerk  SampleTime=-1
      settings: Save2DSignal=2-D array (concatenate along first dimension)
  To Workspace3 : ToWorkspace  VariableName=ax_filt  SampleTime=-1
      settings: Save2DSignal=2-D array (concatenate along first dimension)
  To Workspace4 : ToWorkspace  VariableName=jerk_filt  SampleTime=-1
      settings: Save2DSignal=2-D array (concatenate along first dimension)
  To Workspace5 : ToWorkspace  VariableName=timeVector1  SampleTime=-1
      settings: Save2DSignal=2-D array (concatenate along first dimension)
  Uhat0 : Memory  InitialCondition=init_conditions_data.longSpeed
  state0 : Memory
  uHat : Outport  VectorParamsAs1DForOutWhenUnconnected=off
  wires:
  Gain1/1 -> MATLAB Function/6(uRl)
  Simulation clock/1 -> Delay/1, Sum/1, To Workspace5/1
  Demux2/4 -> Gain3/1  "omega_fl"
  Delay/1 -> Sum/2
  Demux2/1 -> Gain/1  "omega_rr"
  state0/1 -> MATLAB Function/1("s ")
  MATLAB Function/1(s) -> state0/1
  Sum/1 -> MATLAB Function/4(T), Integration time-stamp/1
  Uhat0/1 -> MATLAB Function/2("uHat ")
  IMU signal/1 -> Bus Selector1/1
  Gain3/1 -> MATLAB Function/8(uFl)
  Gain2/1 -> MATLAB Function/7(uFr)
  Gain/1 -> MATLAB Function/5(uRr)
  Demux2/2 -> Gain1/1  "omega_rl"
  Bus Selector1/1 -> Lowpass Filter/1, Derivative/1, To Workspace1/1  "<ax>"
  Demux2/3 -> Gain2/1  "omega_fr"
  Omegas/1 -> Demux2/1
  MATLAB Function/2(uHat) -> To Workspace/1, uHat/1, Uhat0/1
  Derivative/1 -> To Workspace2/1
  Lowpass Filter/1 -> Derivative1/1, MATLAB Function/3(ax), To Workspace3/1
  Derivative1/1 -> To Workspace4/1

== system FullVehicleModel_ABS_ESP/Vehicle/Encoders ==
  omega [m/s] : Inport
  Bus Creator : BusCreator  Inputs=4
  Demux : Demux
  Encoders : Outport  VectorParamsAs1DForOutWhenUnconnected=off
  wires:
  omega [m/s]/1 -> Demux/1
  Demux/1 -> Bus Creator/1  "omega_rr"
  Demux/2 -> Bus Creator/2  "omega_rl"
  Demux/3 -> Bus Creator/3  "omega_fr"
  Demux/4 -> Bus Creator/4  "omega_fl"
  Bus Creator/1 -> Encoders/1

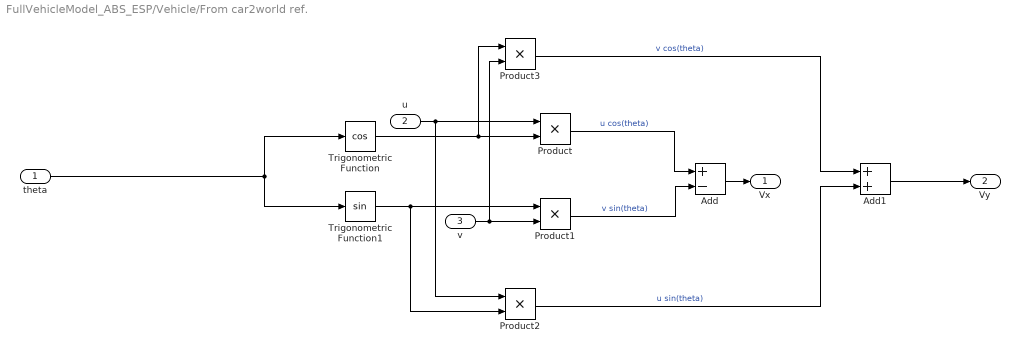
== system FullVehicleModel_ABS_ESP/Vehicle/From car2world ref.  ==
  theta : Inport
  u : Inport  Port=2
  v : Inport  Port=3
  Add : Sum  Inputs=+-
  Add1 : Sum
  Product{,1..3} (4 alike) : Product
  Trigonometric Function : Trigonometry  Operator=cos
  Trigonometric Function1 : Trigonometry
  Vx : Outport  VectorParamsAs1DForOutWhenUnconnected=off
  Vy : Outport  Port=2  VectorParamsAs1DForOutWhenUnconnected=off
  wires:
  theta/1 -> Trigonometric Function/1, Trigonometric Function1/1
  u/1 -> Product/1, Product2/1
  Trigonometric Function/1 -> Product3/1, Product/2
  Trigonometric Function1/1 -> Product1/1, Product2/2
  v/1 -> Product3/2, Product1/2
  Product/1 -> Add/1  "u cos(theta)"
  Product1/1 -> Add/2  "v sin(theta)"
  Add/1 -> Vx/1
  Product3/1 -> Add1/1  "v cos(theta)"
  Add1/1 -> Vy/1
  Product2/1 -> Add1/2  "u sin(theta)"

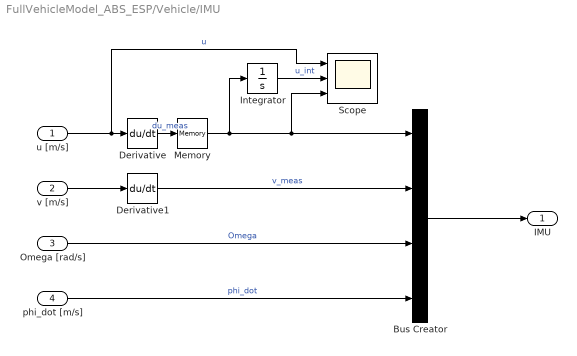
== system FullVehicleModel_ABS_ESP/Vehicle/IMU ==
  u [m/s] : Inport
  v [m/s] : Inport  Port=2
  Omega [rad/s] : Inport  Port=3
  phi_dot [m/s] : Inport  Port=4
  Bus Creator : BusCreator  Inputs=4
  Derivative : Derivative
  Derivative1 : Derivative
  Integrator : Integrator  InitialCondition=V_init/3.6
  Memory : Memory
  Scope : Scope  NumInputPorts=3
  IMU : Outport  VectorParamsAs1DForOutWhenUnconnected=off
  wires:
  u [m/s]/1 -> Derivative/1, Scope/1  "u"
  v [m/s]/1 -> Derivative1/1
  Derivative/1 -> Memory/1  "du_meas"
  Derivative1/1 -> Bus Creator/2  "v_meas"
  Bus Creator/1 -> IMU/1
  Omega [rad/s]/1 -> Bus Creator/3  "Omega"
  phi_dot [m/s]/1 -> Bus Creator/4  "phi_dot"
  Integrator/1 -> Scope/2  "u_int"
  Memory/1 -> Bus Creator/1, Scope/3, Integrator/1

== stateflow chart FullVehicleModel_ABS_ESP/ABS and Wheel torque generation/ABS Rear Left Wheel/ABS Control ==
  state State_q3
    entry: u = 0;
  state State_q2
    entry: u = k;
  state State_q0
    entry: u = -k;
  state State_q1
    entry: u = 0;
  State_q2 -> State_q3 : [Tb >= Tb_max]
  State_q3 -> State_q0 : [lambda >= lambda_max]
  (default) -> State_q0
  State_q1 -> State_q2 : [lambda <= lambda_min]
  State_q0 -> State_q1 : [Tb <= Tb_min]
  data: lambda_min parameter; Tb input; Tb_max parameter; Tb_min parameter; k parameter; lambda input; lambda_max parameter; u output

== stateflow chart FullVehicleModel_ABS_ESP/ABS and Wheel torque generation/ABS Front Right Wheel/ABS Control ==
  state State_q3
    entry: u = 0;
  state State_q2
    entry: u = k;
  state State_q0
    entry: u = -k;
  state State_q1
    entry: u = 0;
  State_q2 -> State_q3 : [Tb >= Tb_max]
  State_q3 -> State_q0 : [lambda >= lambda_max]
  (default) -> State_q0
  State_q1 -> State_q2 : [lambda <= lambda_min]
  State_q0 -> State_q1 : [Tb <= Tb_min]
  data: lambda_min parameter; Tb input; Tb_max parameter; Tb_min parameter; k parameter; lambda input; lambda_max parameter; u output

== stateflow chart FullVehicleModel_ABS_ESP/ABS and Wheel torque generation/ABS Front Left Wheel/ABS Control ==
  state State_q3
    entry: u = 0;
  state State_q2
    entry: u = k;
  state State_q0
    entry: u = -k;
  state State_q1
    entry: u = 0;
  State_q2 -> State_q3 : [Tb >= Tb_max]
  State_q3 -> State_q0 : [lambda >= lambda_max]
  (default) -> State_q0
  State_q1 -> State_q2 : [lambda <= lambda_min]
  State_q0 -> State_q1 : [Tb <= Tb_min]
  data: lambda_min parameter; Tb input; Tb_max parameter; Tb_min parameter; k parameter; lambda input; lambda_max parameter; u output

== matlab function FullVehicleModel_ABS_ESP/ABS and Wheel torque generation/u_estimator/MATLAB Function ==
  data: s input; s output; uHat input; ax input; T input; uRr input; uRl input; uFr input; uFl input; uHat output
function [s,uHat] = lambdaEstimator(s,uHat, ax,T,uRr,uRl,uFr,uFl)
    
    beta  = 0.02*9.81;    % [m/s^2]
    delta = 0.02*9.81;    % [m/s^2]
    uMin = 1;            % [m/s]
    hv = 0.05;
    ha = 0.05;

    
    % compute all the extimations, we suppose RWD 
    uBar = 1/4*(uRr+uRl+uFr+uFl); 
    uND  = 1/2*(uFr+uFl); 

        
    switch round(s)
    case -2
        if uBar <= uMin + hv
            uHat = uBar; 
            s = -2;
        elseif (ax >= delta) && (uBar >= uMin + hv)
            uHat = uND;
            s = -1;
        elseif (ax <= -beta) && (ax >= delta) && (uBar >= uMin + hv)
            uHat = uBar;
            s = 0; 
        elseif (ax <= -beta) && (uBar >= uMin + hv)
            uHat = uHat+ax*T;
            s = 1;
        end
        
    case -1
        if uBar <= uMin
            uHat = uBar; 
            s = -2;
        elseif (ax >= delta) && (uBar > uMin)
            uHat = uND;
            s = -1;
        elseif (ax <= -beta) && (ax >= delta) && (uBar > uMin)
            uHat = uBar;
            s = 0; 
        elseif (ax <= -beta) && (uBar > uMin)
            uHat = uHat+ax*T;
            s = 1;
        end
        
    case 0
        if uBar <= uMin
            uHat = uBar; 
            s = -2;
        elseif (ax >= delta) && (uBar > uMin)
            uHat = uND;
            s = -1;
        elseif (ax <= -beta) && (ax >= delta) && (uBar > uMin)
            uHat = uBar;
            s = 0; 
        elseif (ax <= -beta) && (uBar > uMin)
            uHat = uHat + ax*T;
            s = 1;
        end
        
    case 1
        if uBar <= uMin
            uHat = uBar; 
            s = -2;
        elseif (ax >= delta) && (uBar > uMin)
            uHat = uND;
            s = -1;
        elseif (ax <= -beta + ha) && (ax >= delta) && (uBar > uMin)
            uHat = uBar;
            s = 0; 
        elseif (ax <= -beta + ha) && (uBar > uMin)
            uHat = uHat + ax*T;
            s = 1;
        end
    end
    
end

== stateflow chart FullVehicleModel_ABS_ESP/ABS and Wheel torque generation/ABS Rear Right Wheel/ABS Control ==
  state State_q3
    entry: u = 0;
  state State_q2
    entry: u = k;
  state State_q0
    entry: u = -k;
  state State_q1
    entry: u = 0;
  State_q2 -> State_q3 : [Tb >= Tb_max]
  State_q3 -> State_q0 : [lambda >= lambda_max]
  (default) -> State_q0
  State_q1 -> State_q2 : [lambda <= lambda_min]
  State_q0 -> State_q1 : [Tb <= Tb_min]
  data: lambda_min parameter; Tb input; Tb_max parameter; Tb_min parameter; k parameter; lambda input; lambda_max parameter; u output
